simulink model "GA25_370_130RPM_model"  (R2025b)
settings: Solver=VariableStepAuto  StartTime=0.0  StopTime=20  RelTol=1e-3
model workspace (MAT data in the model file):
  J = 1
  K = Simulink.Parameter
  K.Complexity = 'real'
  K.Dimensions = [0 0]
  K.DataType = 'auto'
  La = Simulink.Parameter
  La.Complexity = 'real'
  La.Dimensions = [0 0]
  La.DataType = 'auto'
  Ra = Simulink.Parameter
  Ra.Complexity = 'real'
  Ra.Dimensions = [0 0]
  Ra.DataType = 'auto'
  b = Simulink.Parameter
  b.Complexity = 'real'
  b.Dimensions = [0 0]
  b.DataType = 'auto'
settings Model: Creator=tarek  LastModifiedBy=Karim
settings DataIOCC: OutputOption=AdditionalOutputTimes  OutputTimes=0:0.01:10  ReturnWorkspaceOutputsName=SDOSimTest_Log

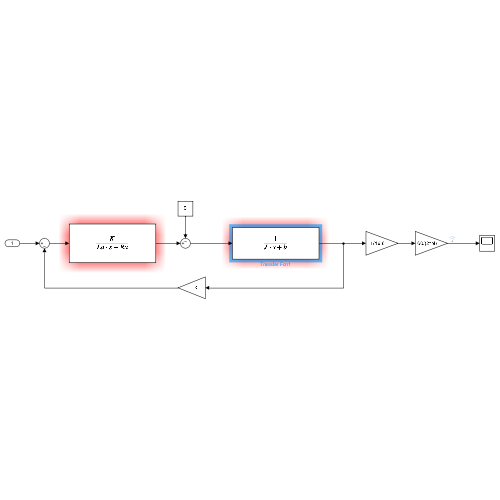
[thumbnail: Simulink's stored preview of the top-level diagram]
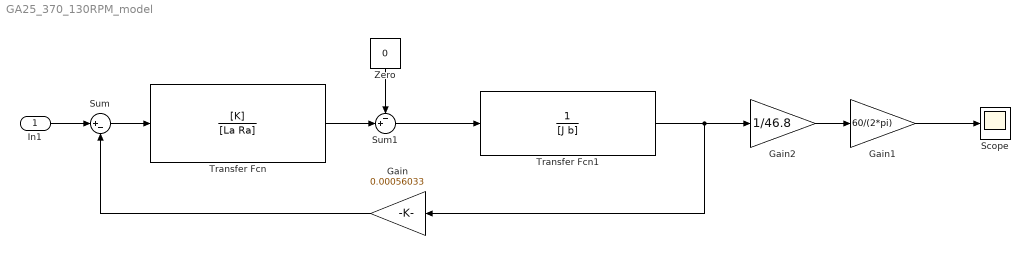
== system GA25_370_130RPM_model ==
  In1 : Inport
  Gain : Gain  Gain=0.00056033
  Gain1 : Gain  Gain=60/(2*pi)
  Gain2 : Gain  Gain=1/46.8
  Scope : Scope
      settings: ActiveDisplayYMinimum=82.398763036578785  ActiveDisplayYMaximum=94.316901298471578
  Sum : Sum  Inputs=|+-
  Sum1 : Sum  Inputs=-+|
  Transfer Fcn : TransferFcn  Numerator=[K]  Denominator=[La Ra]
  Transfer Fcn1 : TransferFcn  Denominator=[J b]
  Zero : Constant  Value=0  OutDataTypeStr=Inherit: Inherit via back propagation
  wires:
  Transfer Fcn/1 -> Sum1/2
  Zero/1 -> Sum1/1
  Sum1/1 -> Transfer Fcn1/1
  Gain/1 -> Sum/2
  Transfer Fcn1/1 -> Gain/1, Gain2/1
  Gain2/1 -> Gain1/1
  Sum/1 -> Transfer Fcn/1
  In1/1 -> Sum/1
  Gain1/1 -> Scope/1
